simulink model "sysgenMRIDemo"  (Simulink 7.7)
settings: Solver=VariableStepDiscrete  StartTime=0.0  StopTime=inf  RelTol=1e-3
PreLoadFcn:
  | sysgenMRIDemo_PreloadFcn
InitFcn:
  | xlFrameDisplay;
undefined symbols (not defined in the file or in its folder): a, b, c_image_cols, c_image_rows, c_num_fstores, c_swathe_size, sysgenMRIDemo_data_imag_channel, xlFrameDisplay
libraries: xbsIndex_r4 x297, dspsrcs4 x3, xbsCopyrightNotice_r4 x1, simulink x1
(part 1 of 3)
settings Model: Creator=arvinds  LastModifiedBy=wayneh

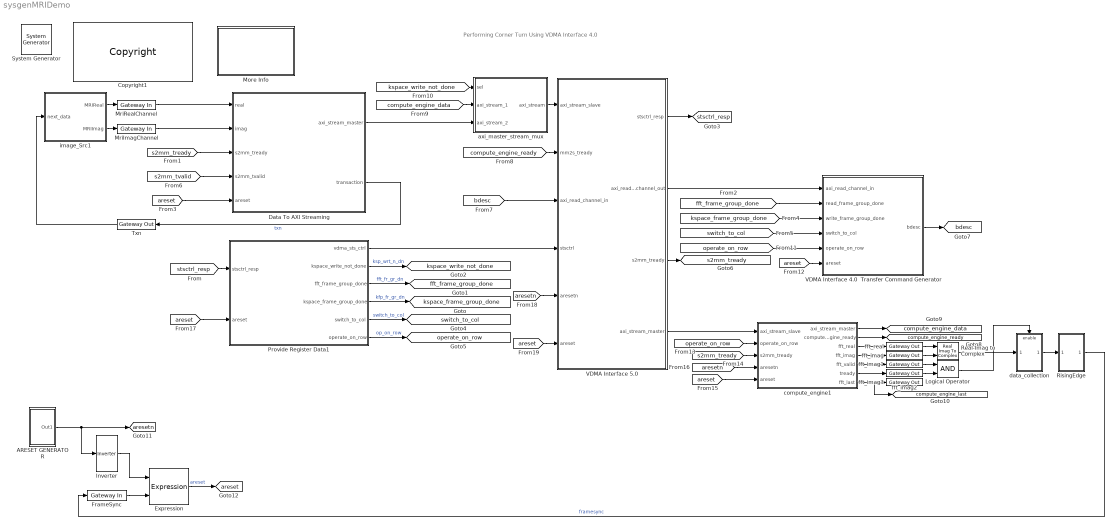
== system sysgenMRIDemo ==
  note: Performing Corner Turn Using VDMA Interface 4.0
  " System Generator" : xbsIndex_r4/ System Generator  Tag=genX  SystemSampleTime=-1  xilinxfamily=virtex6  part=xc6vlx240t  speed=-1  package=ff1156  synthesis_tool=XST  clock_wrapper=Clock Enables  directory=./netlist  proj_type=Project Navigator  Synth_file=XST Defaults  Impl_file=ISE Defaults  testbench=off  simulink_period=1  sysclk_period=10  dcm_input_clock_period=10  incr_netlist=off  trim_vbits=Everywhere in SubSystem  dbl_ovrd=According to Block Masks  core_generation=According to Block Masks  run_coregen=off  deprecated_control=off  eval_field=0  block_type=sysgen
      settings: block_version=12.3
  ARESET GENERATOR : Subsystem
  Copyright1 : xbsCopyrightNotice_r4/Copyright  copyrighttext="Copyright (c) 2011  by  Xilinx, Inc. All rights reserved.<br><br>This file contains proprietary, confidential information of Xilinx, Inc., is distributed under license from Xilinx, Inc., and may be used, copied and/or disclosed only pursuant to the terms of a valid license agreement with Xilinx, Inc. Xilinx hereby grants you a license to use this file solely for design, simulation, implementation and creation of design files limited to Xilinx devices or technologies. Use with non-Xilinx devices or technologies is expressly prohibited and immediately terminates your license unless covered by a separate agreement.<br><br>Xilinx is providing this design, code, or information \"as-is\" solely for use in developing programs and solutions for Xilinx devices, with no obligation on the part of Xilinx to provide support. By providing this design, code, or information as one possible implementation of this feature, application or standard, Xilinx is making no representation that this implementation is free from any claims of infringement. You are responsible for obtaining any rights you may require for your implementation. Xilinx expressly disclaims any warranty whatsoever with respect to the adequacy of the implementation, including but not limited to any warranties or representations that this implementation is free from claims of infringement, implied warranties of merchantability or fitness for a particular purpose.<br><br>Xilinx products are not intended for use in life support appliances, devices, or systems. Use in such applications is expressly prohibited.<br><br>Any modifications that are made to the Source Code are done at the user's sole risk and will be unsupported.<br><br>This copyright and support notice must be retained as part of this text at all times. (c) Copyright 1995-2011 Xilinx, Inc. All rights reserved."  block_type=copyright
      settings: block_version=10.1.00
  Data To AXI Streaming : Subsystem  mask{burst_length=c_image_cols*c_image_cols}
      mask prompts: burst_length "Frame size"
  Expression : xbsIndex_r4/Expression  expression=a | b  align_bp=on  en=off  latency=0  precision=Full  arith_type=Unsigned  n_bits=16  bin_pt=0  dbl_ovrd=off  block_type=expr
      settings: block_version=13.0.2
  FrameSync : xbsIndex_r4/Gateway In  gui_display_data_type=Fixed-point  arith_type=Boolean  n_bits=32  bin_pt=31  preci_type=Single  exp_width=8  frac_width=24  quantization="Round  (unbiased: +/- Inf)"  overflow=Saturate  period=1  dbl_ovrd=off  timing_constraint=None  locs_specified=off  LOCs={}  inherit_from_input=off  UseAsADC=off  ADCChannel='1'  hdl_port=on  block_type=gatewayin
      settings: infoedit="Gateway in block.  Converts inputs of type Simulink integer, double and fixed point to  Xilinx fixed point type.<br><br>Hardware notes:  In hardware these blocks become top level input ports."  block_version=12.2
  Inverter : xbsIndex_r4/Inverter  en=off  latency=0  dbl_ovrd=off  block_type=inv
      settings: block_version=13.0.2
  Logical Operator : Logic  AllPortsSameDT=off  OutDataTypeStr=boolean
  More Info : Subsystem
      mask Display: disp('Double click\n for\n more information.')
  MriImagChannel : xbsIndex_r4/Gateway In  gui_display_data_type=Fixed-point  arith_type="Signed  (2's comp)"  n_bits=32  bin_pt=31  preci_type=Single  exp_width=8  frac_width=24  quantization="Round  (unbiased: +/- Inf)"  overflow=Saturate  period=1  dbl_ovrd=off  timing_constraint=None  locs_specified=off  LOCs={}  inherit_from_input=off  UseAsADC=off  ADCChannel='1'  hdl_port=on  block_type=gatewayin
      settings: infoedit="Gateway in block.  Converts inputs of type Simulink integer, double and fixed point to  Xilinx fixed point type.<br><br>Hardware notes:  In hardware these blocks become top level input ports."  block_version=12.2
  MriRealChannel : xbsIndex_r4/Gateway In  gui_display_data_type=Fixed-point  arith_type="Signed  (2's comp)"  n_bits=32  bin_pt=31  preci_type=Single  exp_width=8  frac_width=24  quantization="Round  (unbiased: +/- Inf)"  overflow=Saturate  period=1  dbl_ovrd=off  timing_constraint=None  locs_specified=off  LOCs={}  inherit_from_input=off  UseAsADC=off  ADCChannel='1'  hdl_port=on  block_type=gatewayin
      settings: infoedit="Gateway in block.  Converts inputs of type Simulink integer, double and fixed point to  Xilinx fixed point type.<br><br>Hardware notes:  In hardware these blocks become top level input ports."  block_version=12.2
  Provide Register Data1 : Subsystem  mask{c_num_frames_to_write=ceil(c_image_rows/c_image_rows), c_num_frames_to_read=ceil(c_image_rows/c_swathe_size), c_num_fstores=c_num_fstores}
      mask prompts: c_num_frames_to_write "Number of frames to write"; c_num_frames_to_read "Number of frames to read"; c_num_fstores "Maximum number of FrameStores"
  Real-Imag to Complex : RealImagToComplex
  RisingEdge : Subsystem
  Txn : xbsIndex_r4/Gateway Out  inherit_from_input=off  hdl_port=on  timing_constraint=None  locs_specified=off  LOCs={}  UseAsDAC=off  DACChannel='1'  block_type=gatewayout
      settings: infoedit="Gateway out block.  Converts Xilinx fixed point inputs into ouputs of type Simulink integer, double, or fixed point.<br><br>Hardware notes:  In hardware these blocks become top level output ports or are discarded, depending on how they are configured."  block_version=12.2
  VDMA Interface 4.0  Transfer Command Generator : Subsystem
  "VDMA Interface 5.0 " : Subsystem
  axi_master_stream_mux : Subsystem
  compute_engine1 : Subsystem
  data_collection : Subsystem
  fft_imag{,1..3} (4 alike) : xbsIndex_r4/Gateway Out  inherit_from_input=off  hdl_port=on  timing_constraint=None  locs_specified=off  LOCs={}  UseAsDAC=off  DACChannel='1'  block_type=gatewayout
      settings: infoedit="Gateway out block.  Converts Xilinx fixed point inputs into ouputs of type Simulink integer, double, or fixed point.<br><br>Hardware notes:  In hardware these blocks become top level output ports or are discarded, depending on how they are configured."  block_version=12.3
  fft_real : xbsIndex_r4/Gateway Out  inherit_from_input=off  hdl_port=on  timing_constraint=None  locs_specified=off  LOCs={}  UseAsDAC=off  DACChannel='1'  block_type=gatewayout
      settings: infoedit="Gateway out block.  Converts Xilinx fixed point inputs into ouputs of type Simulink integer, double, or fixed point.<br><br>Hardware notes:  In hardware these blocks become top level output ports or are discarded, depending on how they are configured."  block_version=12.3
  image_Src1 : Subsystem
  tag scope: areset=global, aresetn=global, bdesc=global, compute_engine_data=global, compute_engine_last=global, compute_engine_ready=global, fft_frame_group_done=global, kspace_frame_group_done=global, kspace_write_not_done=global, operate_on_row=global, s2mm_tready=global, stsctrl_resp=global, switch_to_col=global
  wires:
  MriRealChannel/1 -> Data To AXI Streaming/1(real)
  MriImagChannel/1 -> Data To AXI Streaming/2(imag)
  Data To AXI Streaming/2(transaction) -> Txn/1  "txn"
  [s2mm_tready] -> Data To AXI Streaming/3(s2mm_tready)
  image_Src1/1(MRIReal) -> MriRealChannel/1
  image_Src1/2(MRIImag) -> MriImagChannel/1
  [aresetn] -> "VDMA Interface 5.0 "/5(aresetn)
  Provide Register Data1/1(vdma_sts_ctrl) -> "VDMA Interface 5.0 "/4(stsctrl)
  Provide Register Data1/2(kspace_write_not_done) -> [kspace_write_not_done]  "ksp_wrt_n_dn"
  Provide Register Data1/4(kspace_frame_group_done) -> [kspace_frame_group_done]  "kfp_fr_gr_dn"
  Provide Register Data1/3(fft_frame_group_done) -> [fft_frame_group_done]  "fft_fr_gr_dn"
  "VDMA Interface 5.0 "/2(axi_read_channel_out) -> VDMA Interface 4.0  Transfer Command Generator/1(axi_read_channel_in)
  "VDMA Interface 5.0 "/1(stsctrl_resp) -> [stsctrl_resp]
  [stsctrl_resp] -> Provide Register Data1/1(stsctrl_resp)
  [fft_frame_group_done] -> VDMA Interface 4.0  Transfer Command Generator/2(read_frame_group_done)
  [kspace_frame_group_done] -> VDMA Interface 4.0  Transfer Command Generator/3(write_frame_group_done)
  Provide Register Data1/5(switch_to_col) -> [switch_to_col]  "switch_to_col"
  [switch_to_col] -> VDMA Interface 4.0  Transfer Command Generator/4(switch_to_col)
  Provide Register Data1/6(operate_on_row) -> [operate_on_row]  "op_on_row"
  [operate_on_row] -> VDMA Interface 4.0  Transfer Command Generator/5(operate_on_row)
  "VDMA Interface 5.0 "/3(s2mm_tready) -> [s2mm_tready]
  VDMA Interface 4.0  Transfer Command Generator/1(bdesc) -> [bdesc]
  [bdesc] -> "VDMA Interface 5.0 "/3(axi_read_channel_in)
  compute_engine1/2(compute_engine_ready) -> [compute_engine_ready]
  [compute_engine_ready] -> "VDMA Interface 5.0 "/2(mm2s_tready)
  "VDMA Interface 5.0 "/4(axi_stream_master) -> compute_engine1/1(axi_stream_slave)
  axi_master_stream_mux/1(axi_stream) -> "VDMA Interface 5.0 "/1(axi_stream_slave)
  compute_engine1/1(axi_stream_master) -> [compute_engine_data]
  [kspace_write_not_done] -> axi_master_stream_mux/1(sel)
  Data To AXI Streaming/1(axi_stream_master) -> axi_master_stream_mux/3(axi_stream_2)
  [compute_engine_data] -> axi_master_stream_mux/2(axi_stream_1)
  Txn/1 -> image_Src1/1(next_data)
  compute_engine1/7(fft_last) -> fft_imag3/1, [compute_engine_last]
  ARESET GENERATOR/1(Out1) -> [aresetn], Inverter/1
  [areset] -> Data To AXI Streaming/5(areset)
  [s2mm_tvalid] -> Data To AXI Streaming/4(s2mm_tvalid)
  [areset] -> VDMA Interface 4.0  Transfer Command Generator/6(areset)
  [operate_on_row] -> compute_engine1/2(operate_on_row)
  [s2mm_tready] -> compute_engine1/3(s2mm_tready)
  [areset] -> compute_engine1/5(areset)
  [aresetn] -> compute_engine1/4(aresetn)
  [areset] -> Provide Register Data1/2(areset)
  compute_engine1/3(fft_real) -> fft_real/1
  compute_engine1/4(fft_imag) -> fft_imag/1
  compute_engine1/5(fft_valid) -> fft_imag1/1
  compute_engine1/6(tready) -> fft_imag2/1
  fft_real/1 -> Real-Imag to Complex/1
  fft_imag/1 -> Real-Imag to Complex/2
  fft_imag1/1 -> Logical Operator/1
  fft_imag2/1 -> Logical Operator/2
  Real-Imag to Complex/1 -> data_collection/1(In1)
  Logical Operator/1 -> data_collection/Enable
  FrameSync/1 -> Expression/2
  Inverter/1 -> Expression/1
  Expression/1 -> [areset]  "areset"
  RisingEdge/1(Out1) -> FrameSync/1  "framesync"
  data_collection/1(framesync) -> RisingEdge/1(In1)
  [areset] -> "VDMA Interface 5.0 "/6(areset)

== system sysgenMRIDemo/ARESET GENERATOR ==
  Constant : xbsIndex_r4/Constant  const=31  gui_display_data_type=Fixed-point  arith_type=Unsigned  n_bits=5  bin_pt=0  preci_type=Single  exp_width=8  frac_width=24  explicit_period=off  period=1  equ=P=C  opselect=C  inp2=PCIN>>17  opr=+  inp1=P  carry=CIN  dbl_ovrd=off  block_type=constant
      settings: block_version=13.0.2
  Constant1 : xbsIndex_r4/Constant  const=1  gui_display_data_type=Fixed-point  arith_type=Boolean  n_bits=5  bin_pt=0  preci_type=Single  exp_width=8  frac_width=24  explicit_period=off  period=1  equ=P=C  opselect=C  inp2=PCIN>>17  opr=+  inp1=P  carry=CIN  dbl_ovrd=off  block_type=constant
      settings: block_version=13.0.2
  Counter : xbsIndex_r4/Counter  cnt_type=Free Running  cnt_to=Inf  operation=Up  start_count=0  cnt_by_val=1  arith_type=Unsigned  n_bits=5  bin_pt=0  load_pin=off  rst=off  en=off  explicit_period=on  period=1  dbl_ovrd=off  use_behavioral_HDL=off  implementation=Fabric  block_type=counter
      settings: block_version=13.0.2
  Register : xbsIndex_r4/Register  init=0  rst=off  en=on  dbl_ovrd=off  block_type=register
      settings: block_version=13.0.2
  Relational : xbsIndex_r4/Relational  mode=a=b  en=off  latency=0  dbl_ovrd=off  block_type=relational
      settings: block_version=13.0.2
  Out1 : Outport
  wires:
  Constant1/1 -> Register/1
  Relational/1 -> Register/2
  Constant/1 -> Relational/1
  Counter/1 -> Relational/2
  Register/1 -> Out1/1

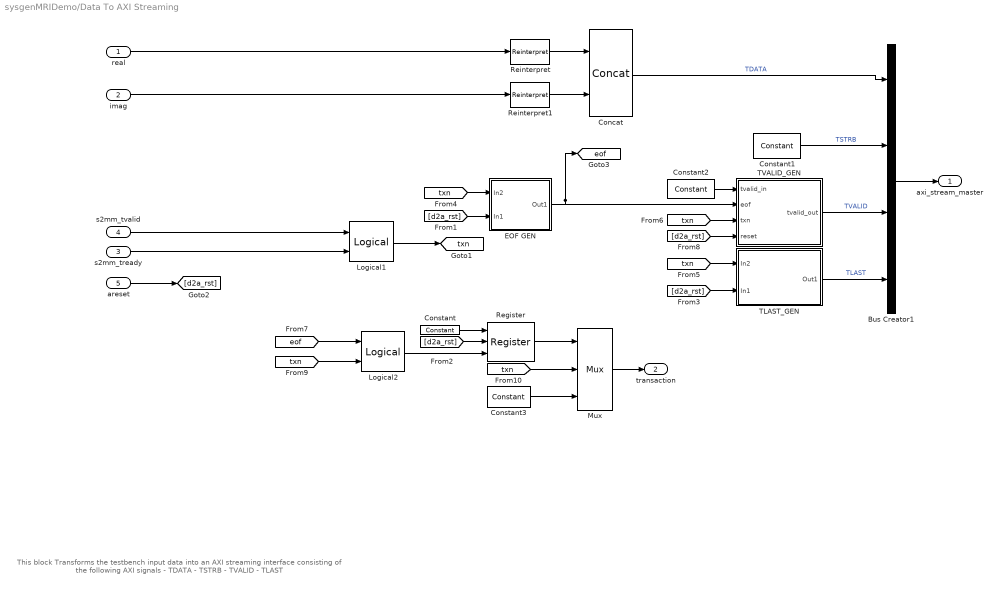
== system sysgenMRIDemo/Data To AXI Streaming ==
  note: This block Transforms the testbench input data into an
      | AXI streaming interface consisting of the following AXI
      | signals
      |   - TDATA
      |   - TSTRB
      |   - TVALID
      |   - TLAST
  real : Inport
  imag : Inport  Port=2
  s2mm_tready : Inport  Port=3
  s2mm_tvalid : Inport  Port=4
  areset : Inport  Port=5
  Bus Creator1 : BusCreator
  Concat : xbsIndex_r4/Concat  num_inputs=2  dbl_ovrd=off  block_type=concat
      settings: block_version=12.3
  Constant : xbsIndex_r4/Constant  const=1  gui_display_data_type=Fixed-point  arith_type=Boolean  n_bits=16  bin_pt=14  preci_type=Single  exp_width=8  frac_width=24  explicit_period=off  period=1  equ=P=C  opselect=C  inp2=PCIN>>17  opr=+  inp1=P  carry=CIN  dbl_ovrd=off  block_type=constant
      settings: block_version=13.0.2
  Constant1 : xbsIndex_r4/Constant  const=2^8-1  gui_display_data_type=Fixed-point  arith_type=Unsigned  n_bits=8  bin_pt=0  preci_type=Single  exp_width=8  frac_width=24  explicit_period=on  period=1  equ=P=C  opselect=C  inp2=PCIN>>17  opr=+  inp1=P  carry=CIN  dbl_ovrd=off  block_type=constant
      settings: block_version=12.3
  Constant2 : xbsIndex_r4/Constant  const=1  gui_display_data_type=Fixed-point  arith_type=Boolean  n_bits=8  bin_pt=0  preci_type=Single  exp_width=8  frac_width=24  explicit_period=on  period=1  equ=P=C  opselect=C  inp2=PCIN>>17  opr=+  inp1=P  carry=CIN  dbl_ovrd=off  block_type=constant
      settings: block_version=12.3
  Constant3 : xbsIndex_r4/Constant  const=0  gui_display_data_type=Fixed-point  arith_type=Boolean  n_bits=16  bin_pt=14  preci_type=Single  exp_width=8  frac_width=24  explicit_period=off  period=1  equ=P=C  opselect=C  inp2=PCIN>>17  opr=+  inp1=P  carry=CIN  dbl_ovrd=off  block_type=constant
      settings: block_version=13.0.2
  EOF GEN : Subsystem
  Logical1 : xbsIndex_r4/Logical  logical_function=AND  inputs=2  en=off  latency=0  precision=Full  arith_type=Unsigned  n_bits=16  bin_pt=0  align_bp=on  dbl_ovrd=off  block_type=logical
      settings: block_version=12.3
  Logical2 : xbsIndex_r4/Logical  logical_function=AND  inputs=2  en=off  latency=0  precision=Full  arith_type=Unsigned  n_bits=16  bin_pt=0  align_bp=on  dbl_ovrd=off  block_type=logical
      settings: block_version=12.3
  Mux : xbsIndex_r4/Mux  inputs=2  en=off  latency=0  precision=Full  arith_type=Unsigned  n_bits=16  bin_pt=14  quantization=Truncate  overflow=Wrap  dbl_ovrd=off  block_type=mux
      settings: block_version=13.0.2
  Register : xbsIndex_r4/Register  init=0  rst=on  en=on  dbl_ovrd=off  block_type=register
      settings: block_version=13.0.2
  Reinterpret : xbsIndex_r4/Reinterpret  force_arith_type=on  arith_type=Unsigned  force_bin_pt=on  bin_pt=0  block_type=reinterpret
      settings: infoedit="Changes signal type without altering the binary representation.   You can changed the signal between signed and unsigned, and relocate the binary point.<br><br>Hardware notes: In hardware this block costs nothing.<br><br>Example:  Suppose the input is 6 bits wide, signed, with 2 fractional bits, and the output is forced to unsigned with 0 fractional bits.  Then an input of -2.0 (1110.00 in binary 2's complement) becomes an output of 56 (111000 in binary)."  block_version=12.3
  Reinterpret1 : xbsIndex_r4/Reinterpret  force_arith_type=on  arith_type=Unsigned  force_bin_pt=on  bin_pt=0  block_type=reinterpret
      settings: infoedit="Changes signal type without altering the binary representation.   You can changed the signal between signed and unsigned, and relocate the binary point.<br><br>Hardware notes: In hardware this block costs nothing.<br><br>Example:  Suppose the input is 6 bits wide, signed, with 2 fractional bits, and the output is forced to unsigned with 0 fractional bits.  Then an input of -2.0 (1110.00 in binary 2's complement) becomes an output of 56 (111000 in binary)."  block_version=12.3
  TLAST_GEN : Subsystem
  TVALID_GEN : Subsystem
  axi_stream_master : Outport
  transaction : Outport  Port=2
  tag scope: eof=global, txn=global
  wires:
  Constant1/1 -> Bus Creator1/2  "TSTRB"
  Bus Creator1/1 -> axi_stream_master/1
  Concat/1 -> Bus Creator1/1  "TDATA"
  s2mm_tready/1 -> Logical1/2
  Logical1/1 -> [txn]
  real/1 -> Reinterpret/1
  imag/1 -> Reinterpret1/1
  s2mm_tvalid/1 -> Logical1/1
  Reinterpret/1 -> Concat/1
  Reinterpret1/1 -> Concat/2
  EOF GEN/1(Out1) -> [eof], TVALID_GEN/2(eof)
  TLAST_GEN/1(Out1) -> Bus Creator1/4  "TLAST"
  Constant2/1 -> TVALID_GEN/1(tvalid_in)
  areset/1 -> [d2a_rst]
  [d2a_rst] -> EOF GEN/2(In1)
  [d2a_rst] -> TLAST_GEN/2(In1)
  [txn] -> EOF GEN/1(In2)
  [txn] -> TLAST_GEN/1(In2)
  TVALID_GEN/1(tvalid_out) -> Bus Creator1/3  "TVALID"
  [txn] -> TVALID_GEN/3(txn)
  [d2a_rst] -> TVALID_GEN/4(reset)
  [d2a_rst] -> Register/2
  Logical2/1 -> Register/3
  [eof] -> Logical2/1
  [txn] -> Logical2/2
  Constant/1 -> Register/1
  Register/1 -> Mux/1
  Mux/1 -> transaction/1
  [txn] -> Mux/2
  Constant3/1 -> Mux/3

== system sysgenMRIDemo/More Info ==
  note: This design implements 2D FFT using a 1D FFT kernel and VDMA Interface 4.0  block. Corner turns for the FFT is performed using the
      | VDMA Interface 4.0  block in System Generator. The VDMA Interface 4.0  is a simulation only block and the block transforms into top level
      | Gateway Ins and Gateway Outs on netlisting. Further use of the design requires stitching it with VDMA IP available in
      | Xilinx Platform Studio.
      |
      | The input data is 256x256 image. The data is first written to external memory as one frame. The data is then read row wise and
      | supplied to the FFT block. Results are overwritten into the external memory through the VDMA interface block. The data is then
      | read column wise from external memory and supplied to the FFT block which produces the resultant 2D FFT.
      |
      | The input to the design is a regridded 2D Kspace image frequently encountered in Magnetic Resonance Imaging Systems(MRI).
      | FFT on this data will result in creating a Sagittal Image of the human head. On loading the design a Figure will be loaded which is
      | the K-Space FFT data and on completing the FFT you will obtain the Sagittal Image of human head. Due to slow simulation speed
      | of the AXI FFT block, it takes ~1 hr for the demo to complete. It is recommended to use HWCosim to speed up the simulation.
      |
      | The design can be netlisted using HDL Netlist in which case the VDMA Interface 4.0  block will be translated into top level gateways.
      | Furthermore, xlVDMACreateProject function can be used to create an ISE project to stitch SysGen design with VDMA Interface 4.0
      | & External Memory in XPS.
      |
      | For more information please type the following in matlab console :
      | >>help xlVDMACreateProject
  note: Performing Corner Turn Using VDMA Interface 4.0

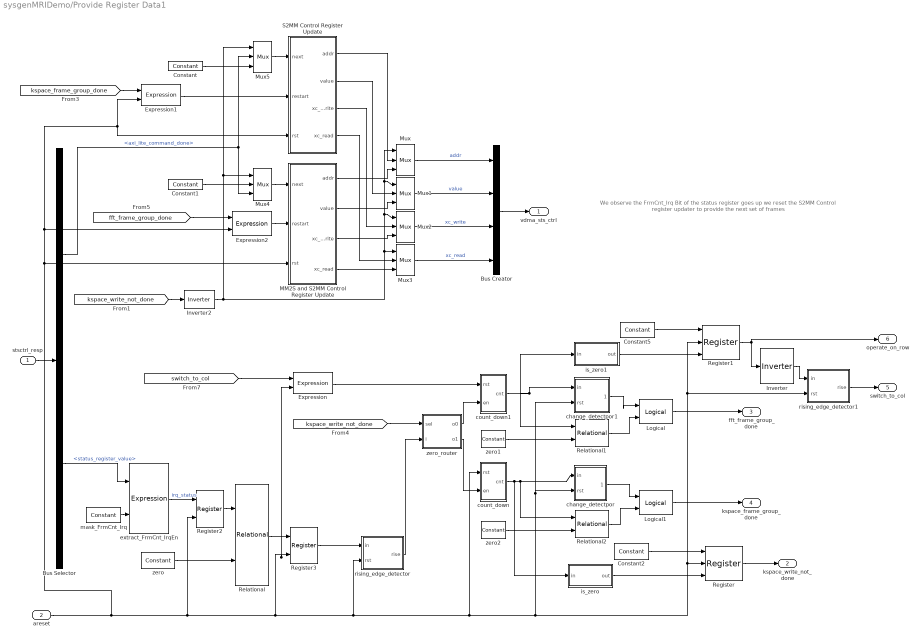
== system sysgenMRIDemo/Provide Register Data1 ==
  note: We observe the FrmCnt_Irq Bit of the status register goes up
      | we reset the S2MM Control register updater to provide the next
      | set of frames
  stsctrl_resp : Inport
  areset : Inport  Port=2
  Bus Creator : BusCreator
  Bus Selector : BusSelector  OutputSignals=axi_lite_command_done,status_register_value
  Constant{,1..2,5} (4 alike) : xbsIndex_r4/Constant  const=0  gui_display_data_type=Fixed-point  arith_type=Boolean  n_bits=16  bin_pt=14  preci_type=Single  exp_width=8  frac_width=24  explicit_period=off  period=1  equ=P=C  opselect=C  inp2=PCIN>>17  opr=+  inp1=P  carry=CIN  dbl_ovrd=off  block_type=constant
      settings: block_version=12.3
  Expression : xbsIndex_r4/Expression  expression=a | b  align_bp=on  en=off  latency=0  precision=Full  arith_type=Unsigned  n_bits=16  bin_pt=0  dbl_ovrd=off  block_type=expr
      settings: block_version=12.3
  Expression1 : xbsIndex_r4/Expression  expression=a | b  align_bp=on  en=off  latency=0  precision=Full  arith_type=Unsigned  n_bits=16  bin_pt=0  dbl_ovrd=off  block_type=expr
      settings: block_version=12.3
  Expression2 : xbsIndex_r4/Expression  expression=a | b  align_bp=on  en=off  latency=0  precision=Full  arith_type=Unsigned  n_bits=16  bin_pt=0  dbl_ovrd=off  block_type=expr
      settings: block_version=12.3
  Inverter : xbsIndex_r4/Inverter  en=off  latency=0  dbl_ovrd=off  block_type=inv
      settings: block_version=12.3
  Inverter2 : xbsIndex_r4/Inverter  en=off  latency=0  dbl_ovrd=off  block_type=inv
      settings: block_version=12.3
  Logical : xbsIndex_r4/Logical  logical_function=AND  inputs=2  en=off  latency=0  precision=Full  arith_type=Unsigned  n_bits=16  bin_pt=0  align_bp=on  dbl_ovrd=off  block_type=logical
      settings: block_version=12.3
  Logical1 : xbsIndex_r4/Logical  logical_function=AND  inputs=2  en=off  latency=0  precision=Full  arith_type=Unsigned  n_bits=16  bin_pt=0  align_bp=on  dbl_ovrd=off  block_type=logical
      settings: block_version=12.3
  MM2S and S2MM Control Register Update : Subsystem
  Mux{,1..5} (6 alike) : xbsIndex_r4/Mux  inputs=2  en=off  latency=0  precision=Full  arith_type=Unsigned  n_bits=16  bin_pt=14  quantization=Truncate  overflow=Wrap  dbl_ovrd=off  block_type=mux
      settings: block_version=12.3
  Register : xbsIndex_r4/Register  init=1  rst=on  en=on  dbl_ovrd=off  block_type=register
      settings: block_version=12.3
  Register1 : xbsIndex_r4/Register  init=1  rst=on  en=on  dbl_ovrd=off  block_type=register
      settings: block_version=12.3
  Register2 : xbsIndex_r4/Register  init=0  rst=on  en=off  dbl_ovrd=off  block_type=register
      settings: block_version=12.3
  Register3 : xbsIndex_r4/Register  init=0  rst=on  en=off  dbl_ovrd=off  block_type=register
      settings: block_version=12.3
  Relational : xbsIndex_r4/Relational  mode=a!=b  en=off  latency=0  dbl_ovrd=off  block_type=relational
      settings: block_version=12.3
  Relational1 : xbsIndex_r4/Relational  mode=a!=b  en=off  latency=0  dbl_ovrd=off  block_type=relational
      settings: block_version=12.3
  Relational2 : xbsIndex_r4/Relational  mode=a!=b  en=off  latency=0  dbl_ovrd=off  block_type=relational
      settings: block_version=12.3
  S2MM Control Register Update : Subsystem
  change_detectpor : Subsystem
  change_detectpor1 : Subsystem
  count_down : Subsystem  mask{init_val=ceil(c_num_frames_to_write / c_num_fstores)}
      mask prompts: init_val "Initial Value"
  count_down1 : Subsystem  mask{init_val=ceil( (c_image_rows/c_swathe_size) / c_num_fstores)}
      mask prompts: init_val "Initial Value"
  extract_FrmCnt_IrqEn : xbsIndex_r4/Expression  expression=a & b  align_bp=on  en=off  latency=0  precision=Full  arith_type=Unsigned  n_bits=16  bin_pt=0  dbl_ovrd=off  block_type=expr
      settings: block_version=12.3
  is_zero : Subsystem
      mask Display: disp('==0')
  is_zero1 : Subsystem
      mask Display: disp('==0')
  mask_FrmCnt_Irq : xbsIndex_r4/Constant  const=hex2dec('00001000')  gui_display_data_type=Fixed-point  arith_type=Signed (2's comp)  n_bits=32  bin_pt=0  preci_type=Single  exp_width=8  frac_width=24  explicit_period=off  period=1  equ=P=C  opselect=C  inp2=PCIN>>17  opr=+  inp1=P  carry=CIN  dbl_ovrd=off  block_type=constant
      settings: block_version=12.3
  rising_edge_detector : Subsystem
      mask Display: disp('\lceil','texmode','on')
  rising_edge_detector1 : Subsystem
      mask Display: disp('\lceil','texmode','on')
  zero : xbsIndex_r4/Constant  const=0  gui_display_data_type=Fixed-point  arith_type=Signed (2's comp)  n_bits=32  bin_pt=0  preci_type=Single  exp_width=8  frac_width=24  explicit_period=off  period=1  equ=P=C  opselect=C  inp2=PCIN>>17  opr=+  inp1=P  carry=CIN  dbl_ovrd=off  block_type=constant
      settings: block_version=12.3
  zero1 : xbsIndex_r4/Constant  const=0  gui_display_data_type=Fixed-point  arith_type=Signed (2's comp)  n_bits=32  bin_pt=0  preci_type=Single  exp_width=8  frac_width=24  explicit_period=off  period=1  equ=P=C  opselect=C  inp2=PCIN>>17  opr=+  inp1=P  carry=CIN  dbl_ovrd=off  block_type=constant
      settings: block_version=12.3
  zero2 : xbsIndex_r4/Constant  const=0  gui_display_data_type=Fixed-point  arith_type=Signed (2's comp)  n_bits=32  bin_pt=0  preci_type=Single  exp_width=8  frac_width=24  explicit_period=off  period=1  equ=P=C  opselect=C  inp2=PCIN>>17  opr=+  inp1=P  carry=CIN  dbl_ovrd=off  block_type=constant
      settings: block_version=12.3
  zero_router : Subsystem
  vdma_sts_ctrl : Outport
  kspace_write_not_done : Outport  Port=2
  fft_frame_group_done : Outport  Port=3
  kspace_frame_group_done : Outport  Port=4
  switch_to_col : Outport  Port=5
  operate_on_row : Outport  Port=6
  wires:
  [fft_frame_group_done] -> Expression2/1
  Inverter/1 -> rising_edge_detector1/1(in)
  Constant5/1 -> Register1/1
  is_zero1/1(out) -> Register1/3
  Register1/1 -> Inverter/1, operate_on_row/1
  Logical1/1 -> kspace_frame_group_done/1
  zero2/1 -> Relational2/2
  Relational2/1 -> Logical1/2
  change_detectpor/1(change) -> Logical1/1
  Relational1/1 -> Logical/2
  zero1/1 -> Relational1/2
  Logical/1 -> fft_frame_group_done/1
  change_detectpor1/1(change) -> Logical/1
  zero_router/1(o0) -> count_down1/2(en)
  zero_router/2(o1) -> count_down/2(en)
  rising_edge_detector/1(rise) -> zero_router/2(i)
  [kspace_write_not_done] -> zero_router/1(sel)
  count_down1/1(cnt) -> is_zero1/1(in), change_detectpor1/1(in), Relational1/1
  is_zero/1(out) -> Register/3
  Register/1 -> kspace_write_not_done/1
  Constant2/1 -> Register/1
  Relational/1 -> Register3/1
  count_down/1(cnt) -> Relational2/1, change_detectpor/1(in), is_zero/1(in)
  [kspace_frame_group_done] -> Expression1/1
  zero/1 -> Relational/2
  extract_FrmCnt_IrqEn/1 -> Register2/1  "irq_status"
  mask_FrmCnt_Irq/1 -> extract_FrmCnt_IrqEn/2
  Bus Selector/2 -> extract_FrmCnt_IrqEn/1  "<status_register_value>"
  Bus Creator/1 -> vdma_sts_ctrl/1
  Mux5/1 -> S2MM Control Register Update/1(next)
  Mux3/1 -> Bus Creator/4  "xc_read"
  Mux2/1 -> Bus Creator/3  "xc_write"
  Mux1/1 -> Bus Creator/2  "value"
  Mux/1 -> Bus Creator/1  "addr"
  [kspace_write_not_done] -> Inverter2/1
  Constant1/1 -> Mux4/2
  Constant/1 -> Mux5/3
  Mux4/1 -> MM2S and S2MM Control Register Update/1(next)
  S2MM Control Register Update/4(xc_read) -> Mux3/2
  S2MM Control Register Update/3(xc_write) -> Mux2/2
  S2MM Control Register Update/2(value) -> Mux1/2
  S2MM Control Register Update/1(addr) -> Mux/2
  Bus Selector/1 -> Mux5/2, Mux4/3  "<axi_lite_command_done>"
  stsctrl_resp/1 -> Bus Selector/1
  rising_edge_detector1/1(rise) -> switch_to_col/1
  Register2/1 -> Relational/1
  Register3/1 -> rising_edge_detector/1(in)
  areset/1 -> Register2/2, rising_edge_detector/2(rst), count_down/1(rst), change_detectpor1/2(rst), change_detectpor/2(rst), Register/2, Register1/2, rising_edge_detector1/2(rst), Register3/2, Expression/2, Expression2/2, Expression1/2, S2MM Control Register Update/3(rst), MM2S and S2MM Control Register Update/3(rst)
  [switch_to_col] -> Expression/1
  Expression/1 -> count_down1/1(rst)
  Expression1/1 -> S2MM Control Register Update/2(restart)
  Expression2/1 -> MM2S and S2MM Control Register Update/2(restart)
  Inverter2/1 -> Mux4/1, Mux5/1, Mux/1, Mux1/1, Mux2/1, Mux3/1
  MM2S and S2MM Control Register Update/1(addr) -> Mux/3
  MM2S and S2MM Control Register Update/2(value) -> Mux1/3
  MM2S and S2MM Control Register Update/3(xc_write) -> Mux2/3
  MM2S and S2MM Control Register Update/4(xc_read) -> Mux3/3

== system sysgenMRIDemo/RisingEdge ==
  In1 : Inport
  Logical Operator1 : Logic  AllPortsSameDT=off  OutDataTypeStr=boolean
  Logical Operator3 : Logic  Operator=NOT  AllPortsSameDT=off  OutDataTypeStr=boolean
  Unit Delay : UnitDelay  SampleTime=-1
  Unit Delay1 : UnitDelay  SampleTime=-1
  Out1 : Outport
  wires:
  In1/1 -> Unit Delay/1, Logical Operator1/1
  Unit Delay/1 -> Logical Operator3/1
  Logical Operator1/1 -> Unit Delay1/1
  Logical Operator3/1 -> Logical Operator1/2
  Unit Delay1/1 -> Out1/1

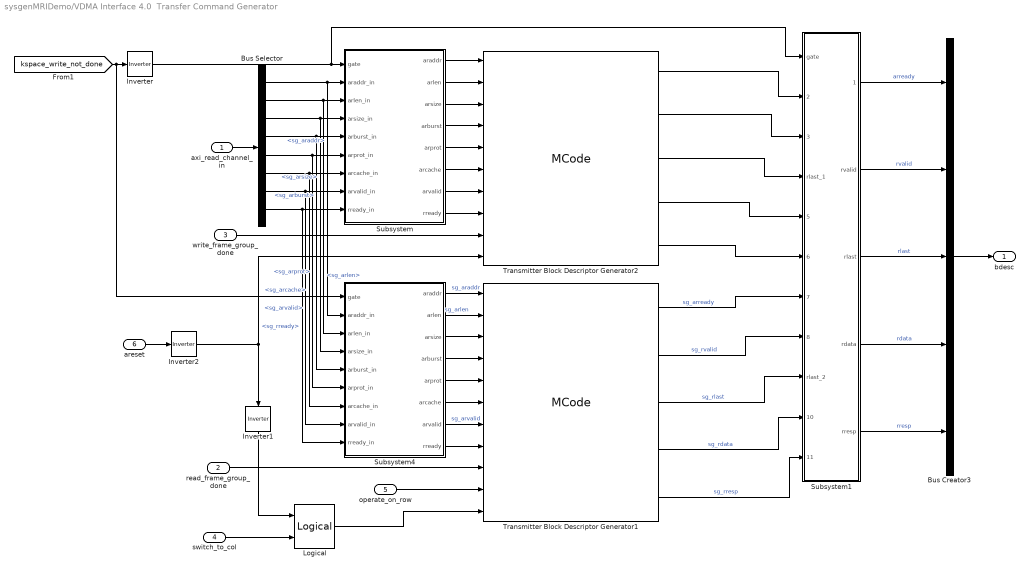
== system sysgenMRIDemo/VDMA Interface 4.0  Transfer Command Generator ==
  axi_read_channel_in : Inport
  read_frame_group_done : Inport  Port=2
  write_frame_group_done : Inport  Port=3
  switch_to_col : Inport  Port=4
  operate_on_row : Inport  Port=5
  areset : Inport  Port=6
  Bus Creator3 : BusCreator  Inputs=5
  Bus Selector : BusSelector  OutputSignals=sg_araddr,sg_arlen,sg_arsize,sg_arburst,sg_arprot,sg_arcache,sg_arvalid,sg_rready
  Inverter : xbsIndex_r4/Inverter  en=off  latency=0  dbl_ovrd=off  block_type=inv
      settings: block_version=12.3
  Inverter1 : xbsIndex_r4/Inverter  en=off  latency=0  dbl_ovrd=off  block_type=inv
      settings: block_version=12.3
  Inverter2 : xbsIndex_r4/Inverter  en=off  latency=0  dbl_ovrd=off  block_type=inv
      settings: block_version=12.3
  Logical : xbsIndex_r4/Logical  logical_function=OR  inputs=2  en=off  latency=0  precision=Full  arith_type=Unsigned  n_bits=16  bin_pt=0  align_bp=on  dbl_ovrd=off  block_type=logical
      settings: block_version=12.3
  Subsystem : Subsystem
  Subsystem1 : Subsystem
  Subsystem4 : Subsystem
  Transmitter Block Descriptor Generator1 : xbsIndex_r4/MCode  mfname=xlScatterGatherEngineLineTransfer2  explicit_period=on  period=1  inputsTable={'boundInpExpr'=>['','','','','','','','','','','','c_image_cols','c_image_rows','c_swathe_size','c_word_size','0','1024'],'inputs'=>['araddr','arlen','arsize','arburst','arprot','arcache','arvalid','rready','resetbd','raster_scan','resetall','IMAGE_COLS','IMAGE_ROWS','SWATHE_SIZE','WORD_SIZE','BANK0_START_ADDRESS','BANK1_START_ADDRESS']}  outputsTable={'outputs'=>['arready','rvalid','rlast','rdata','rresp'],'suppressOut'=>['off','off','off','off','off']}  dbl_ovrd=off  enable_stdout=on  enable_debug=off  suppress_output=on  defparams={'IMAGE_COLS',c_image_cols,'IMAGE_ROWS',c_image_rows,'SWATHE_SIZE',c_swathe_size,'WORD_SIZE',c_word_size,'BANK0_START_ADDRESS',0,'BANK1_START_ADDRESS',1024}  hide_port_list={}  block_type=mcode
      settings: block_version=12.3
  Transmitter Block Descriptor Generator2 : xbsIndex_r4/MCode  mfname=xlScatterGatherEngineLineTransfer  explicit_period=on  period=1  inputsTable={'boundInpExpr'=>['','','','','','','','','','','c_image_cols','c_image_rows','c_image_rows','c_word_size'],'inputs'=>['araddr','arlen','arsize','arburst','arprot','arcache','arvalid','rready','resetbd','aresetn','IMAGE_COLS','IMAGE_ROWS','SWATHE_SIZE','WORD_SIZE']}  outputsTable={'outputs'=>['arready','rvalid','rlast','rdata','rresp'],'suppressOut'=>['off','off','off','off','off']}  dbl_ovrd=off  enable_stdout=on  enable_debug=off  suppress_output=on  defparams={'IMAGE_COLS',c_image_cols,'IMAGE_ROWS',c_image_rows,'SWATHE_SIZE',c_image_rows,'WORD_SIZE',c_word_size}  hide_port_list={}  block_type=mcode
      settings: block_version=12.3
  bdesc : Outport
  wires:
  Logical/1 -> Transmitter Block Descriptor Generator1/11
  areset/1 -> Inverter2/1
  operate_on_row/1 -> Transmitter Block Descriptor Generator1/10
  write_frame_group_done/1 -> Transmitter Block Descriptor Generator2/9
  read_frame_group_done/1 -> Transmitter Block Descriptor Generator1/9
  axi_read_channel_in/1 -> Bus Selector/1
  Bus Creator3/1 -> bdesc/1
  Subsystem1/5(rresp) -> Bus Creator3/5  "rresp"
  Subsystem1/4(rdata) -> Bus Creator3/4  "rdata"
  Subsystem1/3(rlast) -> Bus Creator3/3  "rlast"
  Subsystem1/2(rvalid) -> Bus Creator3/2  "rvalid"
  Subsystem1/1(arready) -> Bus Creator3/1  "arready"
  Transmitter Block Descriptor Generator2/5 -> Subsystem1/6(rresp_1)
  Transmitter Block Descriptor Generator1/5 -> Subsystem1/11(rresp_2)  "sg_rresp"
  Transmitter Block Descriptor Generator1/4 -> Subsystem1/10(rdata_2)  "sg_rdata"
  Transmitter Block Descriptor Generator2/4 -> Subsystem1/5(rdata_1)
  Transmitter Block Descriptor Generator1/3 -> Subsystem1/9(rlast_2)  "sg_rlast"
  Transmitter Block Descriptor Generator2/3 -> Subsystem1/4(rlast_1)
  Transmitter Block Descriptor Generator1/2 -> Subsystem1/8(rvalid_2)  "sg_rvalid"
  Transmitter Block Descriptor Generator2/2 -> Subsystem1/3(rvalid_1)
  Transmitter Block Descriptor Generator1/1 -> Subsystem1/7(arready_2)  "sg_arready"
  Transmitter Block Descriptor Generator2/1 -> Subsystem1/2(arready_1)
  Subsystem4/8(rready) -> Transmitter Block Descriptor Generator1/8
  Subsystem4/7(arvalid) -> Transmitter Block Descriptor Generator1/7  "sg_arvalid"
  Subsystem4/6(arcache) -> Transmitter Block Descriptor Generator1/6
  Subsystem4/5(arprot) -> Transmitter Block Descriptor Generator1/5
  Subsystem4/4(arburst) -> Transmitter Block Descriptor Generator1/4
  Subsystem4/3(arsize) -> Transmitter Block Descriptor Generator1/3
  Subsystem4/2(arlen) -> Transmitter Block Descriptor Generator1/2  "sg_arlen"
  Subsystem4/1(araddr) -> Transmitter Block Descriptor Generator1/1  "sg_araddr"
  Bus Selector/8 -> Subsystem4/9(rready_in), Subsystem/9(rready_in)  "<sg_rready>"
  Bus Selector/7 -> Subsystem4/8(arvalid_in), Subsystem/8(arvalid_in)  "<sg_arvalid>"
  Bus Selector/6 -> Subsystem4/7(arcache_in), Subsystem/7(arcache_in)  "<sg_arcache>"
  Bus Selector/5 -> Subsystem4/6(arprot_in), Subsystem/6(arprot_in)  "<sg_arprot>"
  Bus Selector/4 -> Subsystem4/5(arburst_in), Subsystem/5(arburst_in)  "<sg_arburst>"
  Bus Selector/3 -> Subsystem4/4(arsize_in), Subsystem/4(arsize_in)  "<sg_arsize>"
  Bus Selector/2 -> Subsystem4/3(arlen_in), Subsystem/3(arlen_in)  "<sg_arlen>"
  Bus Selector/1 -> Subsystem4/2(araddr_in), Subsystem/2(araddr_in)  "<sg_araddr>"
  Subsystem/8(rready) -> Transmitter Block Descriptor Generator2/8
  Subsystem/7(arvalid) -> Transmitter Block Descriptor Generator2/7
  Subsystem/6(arcache) -> Transmitter Block Descriptor Generator2/6
  Subsystem/5(arprot) -> Transmitter Block Descriptor Generator2/5
  Subsystem/4(arburst) -> Transmitter Block Descriptor Generator2/4
  Subsystem/3(arsize) -> Transmitter Block Descriptor Generator2/3
  Subsystem/2(arlen) -> Transmitter Block Descriptor Generator2/2
  Subsystem/1(araddr) -> Transmitter Block Descriptor Generator2/1
  [kspace_write_not_done] -> Inverter/1, Subsystem4/1(gate)
  switch_to_col/1 -> Logical/2
  Inverter/1 -> Subsystem/1(gate), Subsystem1/1(gate)
  Inverter2/1 -> Transmitter Block Descriptor Generator2/10, Inverter1/1
  Inverter1/1 -> Logical/1

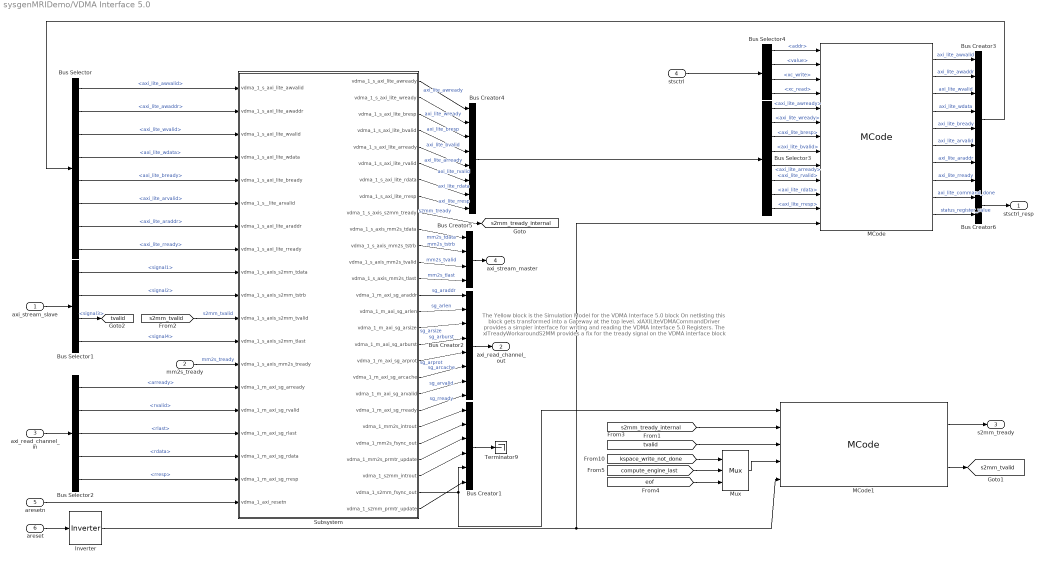
== system sysgenMRIDemo/VDMA Interface 5.0  ==
  note: The Yellow block is the Simulation Model for the VDMA Interface 5.0  block
      | On netlisting this block gets transformed into a Gateway at the top level.
      | xlAXILiteVDMACommandDriver provides a simpler interface for writing
      | and reading the VDMA Interface 5.0  Registers.
      | The xlTreadyWorkaroundS2MM provides a fix for the tready signal on the
      | VDMA interface block
  axi_stream_slave : Inport
  mm2s_tready : Inport  Port=2
  axi_read_channel_in : Inport  Port=3
  stsctrl : Inport  Port=4
  aresetn : Inport  Port=5
  areset : Inport  Port=6
  Bus Creator1 : BusCreator  Inputs=6
  Bus Creator2 : BusCreator  Inputs=8
  Bus Creator3 : BusCreator  Inputs=8
  Bus Creator4 : BusCreator  Inputs=8
  Bus Creator5 : BusCreator
  Bus Creator6 : BusCreator  Inputs=2
  Bus Selector : BusSelector  OutputSignals=axi_lite_awvalid,axi_lite_awaddr,axi_lite_wvalid,axi_lite_wdata,axi_lite_bready,axi_lite_arvalid,axi_lite_araddr,axi_lite_rready
  Bus Selector1 : BusSelector  OutputSignals=signal1,signal2,signal3,signal4
  Bus Selector2 : BusSelector  OutputSignals=arready,rvalid,rlast,rdata,rresp
  Bus Selector3 : BusSelector  OutputSignals=axi_lite_awready,axi_lite_wready,axi_lite_bresp,axi_lite_bvalid,axi_lite_arready,axi_lite_rvalid,axi_lite_rdata,axi_lite_rresp
  Bus Selector4 : BusSelector  OutputSignals=addr,value,xc_write,xc_read
  Inverter : xbsIndex_r4/Inverter  en=off  latency=0  dbl_ovrd=off  block_type=inv
      settings: block_version=13.0.2
  MCode : xbsIndex_r4/MCode  mfname=xlAXILiteVDMACommandDriver  explicit_period=off  period=1  inputsTable={'boundInpExpr'=>['','','','','','','','','','','',''],'inputs'=>['addr','value','xc_write','xc_read','awready','wready','bresp','bvalid','arready','rvalid','rdata','rresp']}  outputsTable={'outputs'=>['awvalid','awaddr','wvalid','wdata','bready','arvalid','araddr','rready','done','read_value'],'suppressOut'=>['off','off','off','off','off','off','off','off','off','off']}  dbl_ovrd=off  enable_stdout=off  enable_debug=off  suppress_output=on  defparams={}  hide_port_list={}  block_type=mcode
      settings: block_version=12.3
  MCode1 : xbsIndex_r4/MCode  mfname=xlTreadyWorkaroundS2MM  explicit_period=off  period=1  inputsTable={'boundInpExpr'=>['','','','','','c_swathe_size'],'inputs'=>['s2mm_fsync_out','s2mm_tready','tvalid','s2mm_tlast','aresetn','VSIZE']}  outputsTable={'outputs'=>['tready','s2mm_tvalid'],'suppressOut'=>['off','off']}  dbl_ovrd=off  enable_stdout=off  enable_debug=off  suppress_output=on  defparams={'VSIZE',c_swathe_size}  hide_port_list={}  block_type=mcode
      settings: block_version=12.3
  Mux : xbsIndex_r4/Mux  inputs=2  en=off  latency=0  precision=Full  arith_type=Unsigned  n_bits=16  bin_pt=14  quantization=Truncate  overflow=Wrap  dbl_ovrd=off  block_type=mux
      settings: block_version=12.3
  Subsystem : Subsystem
  Terminator9 : Terminator
  stsctrl_resp : Outport
  axi_read_channel_out : Outport  Port=2
  s2mm_tready : Outport  Port=3
  axi_stream_master : Outport  Port=4
  tag scope: s2mm_tready_internal=global, s2mm_tvalid=global, tvalid=global
  wires:
  Bus Selector/2 -> Subsystem/2(vdma_1_s_axi_lite_awaddr)  "<axi_lite_awaddr>"
  Bus Selector/3 -> Subsystem/3(vdma_1_s_axi_lite_wvalid)  "<axi_lite_wvalid>"
  Bus Selector/4 -> Subsystem/4(vdma_1_s_axi_lite_wdata)  "<axi_lite_wdata>"
  Bus Selector/5 -> Subsystem/5(vdma_1_s_axi_lite_bready)  "<axi_lite_bready>"
  Bus Selector/6 -> Subsystem/6(vdma_1_s__lite_arvalid)  "<axi_lite_arvalid>"
  Bus Selector/7 -> Subsystem/7(vdma_1_s_axi_lite_araddr)  "<axi_lite_araddr>"
  Bus Selector/8 -> Subsystem/8(vdma_1_s_axi_lite_rready)  "<axi_lite_rready>"
  Subsystem/14(vdma_1_m_axi_sg_araddr) -> Bus Creator2/1  "sg_araddr"
  Subsystem/15(vdma_1_m_axi_sg_arlen) -> Bus Creator2/2  "sg_arlen"
  Subsystem/16(vdma_1_m_axi_sg_arsize) -> Bus Creator2/3  "sg_arsize"
  Subsystem/17(vdma_1_m_axi_sg_arburst) -> Bus Creator2/4  "sg_arburst"
  Subsystem/18(vdma_1_m_axi_sg_arprot) -> Bus Creator2/5  "sg_arprot"
  Subsystem/19(vdma_1_m_axi_sg_arcache) -> Bus Creator2/6  "sg_arcache"
  Subsystem/20(vdma_1_m_axi_sg_arvalid) -> Bus Creator2/7  "sg_arvalid"
  Subsystem/21(vdma_1_m_axi_sg_rready) -> Bus Creator2/8  "sg_rready"
  Bus Selector1/1 -> Subsystem/9(vdma_1_s_axis_s2mm_tdata)  "<signal1>"
  Bus Selector1/2 -> Subsystem/10(vdma_1_s_axis_s2mm_tstrb)  "<signal2>"
  mm2s_tready/1 -> Subsystem/13(vdma_1_s_axis_mm2s_tready)  "mm2s_tready"
  axi_read_channel_in/1 -> Bus Selector2/1
  axi_stream_slave/1 -> Bus Selector1/1
  Subsystem/22(vdma_1_mm2s_introut) -> Bus Creator1/1
  Subsystem/23(vdma_1_mm2s_fsync_out) -> Bus Creator1/2
  Subsystem/24(vdma_1_mm2s_prmtr_update) -> Bus Creator1/3
  Subsystem/25(vdma_1_s2mm_introut) -> Bus Creator1/4
  Bus Creator1/1 -> Terminator9/1
  Subsystem/26(vdma_1_s2mm_fsync_out) -> Bus Creator1/5, MCode1/1
  Subsystem/27(vdma_1_s2mm_prmtr_update) -> Bus Creator1/6
  Bus Selector/1 -> Subsystem/1(vdma_1_s_axi_lite_awvalid)  "<axi_lite_awvalid>"
  MCode/1 -> Bus Creator3/1  "axi_lite_awvalid"
  MCode/2 -> Bus Creator3/2  "axi_lite_awaddr"
  MCode/3 -> Bus Creator3/3  "axi_lite_wvalid"
  MCode/4 -> Bus Creator3/4  "axi_lite_wdata"
  MCode/5 -> Bus Creator3/5  "axi_lite_bready"
  MCode/6 -> Bus Creator3/6  "axi_lite_arvalid"
  MCode/7 -> Bus Creator3/7  "axi_lite_araddr"
  MCode/8 -> Bus Creator3/8  "axi_lite_rready"
  Bus Creator3/1 -> Bus Selector/1
  aresetn/1 -> Subsystem/19(vdma_1_axi_resetn)
  Bus Creator2/1 -> axi_read_channel_out/1
  Subsystem/10(vdma_1_s_axis_mm2s_tdata) -> Bus Creator5/1  "mm2s_tdata"
  Subsystem/11(vdma_1_s_axis_mm2s_tstrb) -> Bus Creator5/2  "mm2s_tstrb"
  Subsystem/12(vdma_1_s_axis_mm2s_tvalid) -> Bus Creator5/3  "mm2s_tvalid"
  Subsystem/13(vdma_1_s_axis_mm2s_tlast) -> Bus Creator5/4  "mm2s_tlast"
  MCode1/1 -> s2mm_tready/1
  [s2mm_tready_internal] -> MCode1/2
  Subsystem/9(vdma_1_s_axis_s2mm_tready) -> [s2mm_tready_internal]  "s2mm_tready"
  MCode1/2 -> [s2mm_tvalid]
  [s2mm_tvalid] -> Subsystem/11(vdma_1_s_axis_s2mm_tvalid)  "s2mm_tvalid"
  Bus Selector1/3 -> [tvalid]  "<signal3>"
  [tvalid] -> MCode1/3
  Bus Selector1/4 -> Subsystem/12(vdma_1_s_axis_s2mm_tlast)  "<signal4>"
  Subsystem/1(vdma_1_s_axi_lite_awready) -> Bus Creator4/1  "axi_lite_awready"
  Subsystem/2(vdma_1_s_axi_lite_wready) -> Bus Creator4/2  "axi_lite_wready"
  Subsystem/3(vdma_1_s_axi_lite_bresp) -> Bus Creator4/3  "axi_lite_bresp"
  Subsystem/4(vdma_1_s_axi_lite_bvalid) -> Bus Creator4/4  "axi_lite_bvalid"
  Subsystem/5(vdma_1_s_axi_lite_arready) -> Bus Creator4/5  "axi_lite_arready"
  Subsystem/6(vdma_1_s_axi_lite_rvalid) -> Bus Creator4/6  "axi_lite_rvalid"
  Subsystem/7(vdma_1_s_axi_lite_rdata) -> Bus Creator4/7  "axi_lite_rdata"
  Subsystem/8(vdma_1_s_axi_lite_rresp) -> Bus Creator4/8  "axi_lite_rresp"
  Bus Selector3/1 -> MCode/5  "<axi_lite_awready>"
  Bus Selector3/2 -> MCode/6  "<axi_lite_wready>"
  Bus Selector3/3 -> MCode/7  "<axi_lite_bresp>"
  Bus Selector3/4 -> MCode/8  "<axi_lite_bvalid>"
  Bus Selector3/5 -> MCode/9  "<axi_lite_arready>"
  Bus Selector3/6 -> MCode/10  "<axi_lite_rvalid>"
  Bus Selector3/7 -> MCode/11  "<axi_lite_rdata>"
  Bus Selector3/8 -> MCode/12  "<axi_lite_rresp>"
  Bus Creator4/1 -> Bus Selector3/1
  Bus Selector4/1 -> MCode/1  "<addr>"
  Bus Selector4/2 -> MCode/2  "<value>"
  Bus Selector4/3 -> MCode/3  "<xc_write>"
  Bus Selector4/4 -> MCode/4  "<xc_read>"
  stsctrl/1 -> Bus Selector4/1
  Bus Creator5/1 -> axi_stream_master/1
  MCode/10 -> Bus Creator6/2  "status_register_value"
  MCode/9 -> Bus Creator6/1  "axi_lite_command_done"
  Bus Creator6/1 -> stsctrl_resp/1
  Bus Selector2/1 -> Subsystem/14(vdma_1_m_axi_sg_arready)  "<arready>"
  Bus Selector2/2 -> Subsystem/15(vdma_1_m_axi_sg_rvalid)  "<rvalid>"
  Bus Selector2/3 -> Subsystem/16(vdma_1_m_axi_sg_rlast)  "<rlast>"
  Bus Selector2/4 -> Subsystem/17(vdma_1_m_axi_sg_rdata)  "<rdata>"
  Bus Selector2/5 -> Subsystem/18(vdma_1_m_axi_sg_rresp)  "<rresp>"
  [eof] -> Mux/3
  [compute_engine_last] -> Mux/2
  [kspace_write_not_done] -> Mux/1
  Mux/1 -> MCode1/4
  areset/1 -> Inverter/1
  Inverter/1 -> MCode1/5, MCode/13

== system sysgenMRIDemo/axi_master_stream_mux ==
  sel : Inport
  axi_stream_1 : Inport  Port=2
  axi_stream_2 : Inport  Port=3
  Bus Creator5 : BusCreator
  Bus Selector : BusSelector  OutputSignals=TDATA,TSTRB,TVALID,TLAST
  Bus Selector1 : BusSelector  OutputSignals=signal1,signal2,signal3,signal4
  Constant : xbsIndex_r4/Constant  const=0  gui_display_data_type=Fixed-point  arith_type=Boolean  n_bits=16  bin_pt=14  preci_type=Single  exp_width=8  frac_width=24  explicit_period=off  period=1  equ=P=C  opselect=C  inp2=PCIN>>17  opr=+  inp1=P  carry=CIN  dbl_ovrd=off  block_type=constant
      settings: block_version=13.0.2
  Mux{,1..5} (6 alike) : xbsIndex_r4/Mux  inputs=2  en=off  latency=0  precision=Full  arith_type=Unsigned  n_bits=16  bin_pt=14  quantization=Truncate  overflow=Wrap  dbl_ovrd=off  block_type=mux
      settings: block_version=12.3
  axi_stream : Outport
  wires:
  Bus Creator5/1 -> axi_stream/1
  Mux3/1 -> Bus Creator5/4
  Mux2/1 -> Bus Creator5/3
  Mux1/1 -> Bus Creator5/2
  Mux/1 -> Bus Creator5/1
  Bus Selector/4 -> Mux3/3  "<TLAST>"
  Bus Selector/3 -> Mux2/3  "<TVALID>"
  Bus Selector/2 -> Mux1/3  "<TSTRB>"
  Bus Selector/1 -> Mux/3  "<TDATA>"
  Bus Selector1/2 -> Mux1/2  "<signal2>"
  Bus Selector1/1 -> Mux/2  "<signal1>"
  sel/1 -> Mux/1, Mux1/1, Mux2/1, Mux3/1
  axi_stream_2/1 -> Bus Selector/1
  axi_stream_1/1 -> Bus Selector1/1
  [operate_on_row] -> Mux4/1
  Mux4/1 -> Mux3/2
  Bus Selector1/4 -> Mux4/3  "<signal4>"
  [operate_on_row] -> Mux5/1
  Bus Selector1/3 -> Mux5/3, Mux4/2  "<signal3>"
  Mux5/1 -> Mux2/2
  Constant/1 -> Mux5/2
